simulink model "merginglines"  (R2021a)
settings: Solver=VariableStepAuto  StartTime=0.0  StopTime=10.0  RelTol=1e-3
settings Model: Creator=ibirl  LastModifiedBy=zht

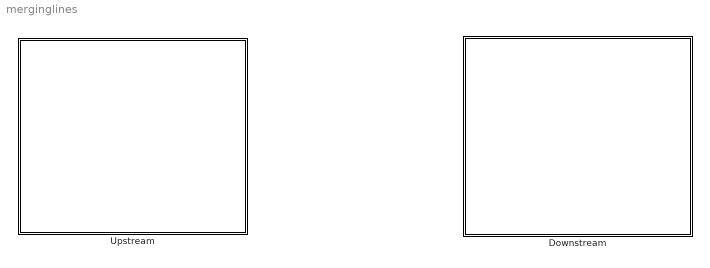
== system merginglines ==
  Downstream : Stateflow chart  TreatAsAtomicUnit=on
  Upstream : Stateflow chart  TreatAsAtomicUnit=on

== stateflow chart merginglines/Downstream ==
  state D1
  state D2
  state D3
  state D4
  D1 -> D1 [order 3] : (1)[1-r3]{0}
  D4 -> D1 [order 2] : (1)[p3]{0}
  D1 -> D3 [order 1] : (1)[r3*pb]{-1}
  D1 -> D2 [order 2] : (1)[r3*(1-pb)]{-1}
  D2 -> D1 [order 2] : (0)[p3*(1-pb)]{0}
  D2 -> D2 [order 3] : (1)[(1-p3)*(1-pb)]{-1}
  D4 -> D2 [order 3] : (1)[(1-p3)*(1-pb)]{-1}
  D2 -> D3 [order 1] : (0)[pb]{-1}
  D3 -> D3 [order 2] : (1)[pbd]{0}
  D3 -> D4 [order 1] : (1)[1-pbd]{0}
  D4 -> D3 [order 1] : (1)[(1-p3)*pb]{-1}

== stateflow chart merginglines/Upstream ==
  state a21
  state a11
  state a31
  state a41
  state a12
  state a22
  state a32
  state a42
  state a33
  state a23
  state a43
  state a13
  state a44
  state a14
  state a24
  state a34
  a41 -> a11 [order 1] : (1)[(p1)*(1-ps1)*(1-r2)]{0}
  a11 -> a31 [order 6] : (1)[r1*ps1*(1-r2)]{1}
  a41 -> a21 [order 5] : (1)[(1-p1)*(1-ps1)*(1-r2)]{1}
  a21 -> a21 [order 5] : (1)[(1-p1)*(1-ps1)*(1-r2)]{1}
  a11 -> a11 [order 1] : (1)[(1-r1)*(1-r2)]{0}
  a21 -> a23 [order 8] : (1)[(1-p1)*(1-ps1)*(r2)*(ps2)]{2}
  a31 -> a31 [order 1] : (1)[(psu1)*(1-r2)]{0}
  a21 -> a11 [order 1] : (1)[p1*(1-ps1)*(1-r2)]{0}
  a21 -> a33 [order 3] : (1)[(1-p1)*ps1*r2*ps2]{2}
  a21 -> a32 [order 9] : (1)[(1-p1)*(ps1)*(r2)*(1-ps2)]{2}
  a21 -> a12 [order 4] : (1)[p1*(1-ps1)*r2*(1-ps2)]{1}
  a22 -> a21 [order 4] : (1)[p1*(1-ps1)*(1-p2)*(1-ps2)]{1}
  a44 -> a11 [order 1] : (1)[(p1)*(1-ps1)*(p2)*(1-ps2)]{0}
  a21 -> a31 [order 7] : (1)[(1-p1)*(ps1)*(1-r2)]{1}
  a31 -> a33 [order 3] : (1)[(psu1)*(r2)*(ps2)]{1}
  a11 -> a21 [order 4] : (1)[r1*(1-ps1)*(1-r2)]{1}
  a14 -> a21 [order 5] : (1)[(r1)*(1-ps1)*(p2)*(1-ps2)]{1}
  a42 -> a21 [order 5] : (1)[(1-p1)*(1-ps1)*(1-r2)]{1}
  a42 -> a11 [order 1] : (1)[(p1)*(1-ps1)*(1-r2)]{0}
  a14 -> a31 [order 7] : (1)[(r1)*(ps1)*(p2)*(1-ps2)]{1}
  a24 -> a31 [order 7] : (1)[(r1)*(ps1)*(p2)*(1-ps2)]{1}
  a44 -> a31 [order 7] : (1)[(1-p1)*(ps1)*(p2)*(1-ps2)]{1}
  a41 -> a23 [order 8] : (1)[(1-p1)*(1-ps1)*(r2)*(ps2)]{2}
  a21 -> a22 [order 2] : (1)[(1-p1)*(1-ps1)*r2*(1-ps2)]{2}
  a12 -> a21 [order 5] : (1)[(r1)*(1-ps1)*(p2)*(1-ps2)]{1}
  a21 -> a13 [order 6] : (1)[(p1)*(1-ps1)*(r2)*(ps2)
      | ]{1}
  a24 -> a21 [order 5] : (1)[(r1)*(1-ps1)*(p2)*(1-ps2)]{1}
  a44 -> a21 [order 5] : (1)[(1-p1)*(1-ps1)*(p2)*(1-ps2)]{1}
  a14 -> a11 [order 1] : (1)[(1-r1)*(p2)*(1-ps2)]{0}
  a31 -> a41 [order 4] : (1)[(1-ppsu1)*(1-r2)]{0}
  a42 -> a31 [order 7] : (1)[(1-p1)*(ps1)*(1-r2)]{1}
  a22 -> a11 [order 1] : (1)[p1*(1-ps1)*p2*(1-ps2)]{0}
  a11 -> a22 [order 2] : (1)[r1*(1-ps1)*r2*(1-ps2)]{2}
  a11 -> a13 [order 5] : (1)[(1-r1)*r2*ps2]{1}
  a24 -> a11 [order 1] : (1)[(1-r1)*(p2)*(1-ps2)]{0}
  a11 -> a12 [order 9] : (1)[(1-r1)*r2*(1-ps2)]{1}
  a11 -> a32 [order 7] : (1)[r1*ps1*r2*(1-ps2)]{2}
  a11 -> a33 [order 3] : (1)[r1*ps1*r2*ps2]{2}
  a11 -> a23 [order 8] : (1)[r1*(1-ps1)*r2*ps2]{2}
  a12 -> a11 [order 1] : (1)[(1-r1)*(p2)*(1-ps2)]{0}
  a12 -> a31 [order 7] : (1)[(r1)*(ps1)*(p2)*(1-ps2)]{1}
  a22 -> a31 [order 8] : (1)[ps1*p2*(1-ps2)]{0}
  a34 -> a31 [order 1] : (1)[(psu1)*(p2)*(1-ps2)]{0}
  a31 -> a42 [order 5] : (1)[(1-ppsu1)*(r2)*(1-ps2)]{1}
  a32 -> a31 [order 1] : (1)[(psu1)*(p2)*(1-ps2)]{0}
  a31 -> a32 [order 2] : (1)[(psu1)*(r2)*(1-ps2)]{1}
  a31 -> a43 [order 6] : (1)[(1-ppsu1)*(r2)*(ps2)]{1}
  a41 -> a31 [order 7] : (1)[(1-p1)*(ps1)*(1-r2)]{1}
  a34 -> a41 [order 4] : (1)[(1-psu1)*(p2)*(1-ps2)]{0}
  a41 -> a12 [order 4] : (1)[(p1)*(1-ps1)*(r2)*(1-ps2)]{1}
  a41 -> a13 [order 6] : (1)[(p1)*(1-ps1)*(r2)*(ps2)]{1}
  a41 -> a22 [order 2] : (1)[(1-p1)*(1-ps1)*(r2)*(1-ps2)]{2}
  a41 -> a33 [order 3] : (1)[(1-p1)*(ps1)*(r2)*(ps2)]{2}
  a32 -> a41 [order 4] : (1)[(1-ppsu1)*(p2)*(1-ps2)]{0}
  a41 -> a32 [order 9] : (1)[(1-p1)*(ps1)*(r2)*(1-ps2)]{2}
  a22 -> a12 [order 5] : (1)[(1-p1)*(1-ps1)*p2*(1-ps2)]{1}
  a12 -> a12 [order 4] : (1)[(1-r1)*(1-p2)*(1-ps2)]{1}
  a12 -> a13 [order 6] : (1)[(1-r1)*(1-p2)*(ps2)]{1}
  a44 -> a12 [order 4] : (1)[(p1)*(1-ps1)*(1-p2)*(1-ps2)]{1}
  a14 -> a12 [order 4] : (1)[(1-r1)*(1-p2)*(1-ps2)]{1}
  a42 -> a22 [order 2] : (1)[(1-p1)*(1-ps1)*(r2)*(1-ps2)]{2}
  a24 -> a12 [order 4] : (1)[(1-r1)*(1-p2)*(1-ps2)]{1}
  a12 -> a33 [order 3] : (1)[(r1)*(ps1)*(1-p2)*(ps2)]{2}
  a12 -> a32 [order 9] : (1)[(r1)*(ps1)*(1-p2)*(1-ps2)]{2}
  a12 -> a22 [order 2] : (1)[(r1)*(1-ps1)*(1-p2)*(1-ps2)]{2}
  a12 -> a23 [order 8] : (1)[(r1)*(1-ps1)*(1-p2)*(ps2)]{2}
  a42 -> a12 [order 4] : (1)[(p1)*(1-ps1)*(r2)*(1-ps2)]{1}
  a32 -> a32 [order 2] : (1)[(psu1)*(1-p2)*(1-ps2)]{1}
  a22 -> a22 [order 2] : (1)[(1-p1)*(1-ps1)*(1-p2)*(1-ps2)]{2}
  a22 -> a32 [order 6] : (1)[ps1*(1-p2)*(1-ps2)]{2}
  a14 -> a22 [order 2] : (1)[(r1)*(1-ps1)*(1-p2)*(1-ps2)]{2}
  a14 -> a32 [order 9] : (1)[(r1)*(ps1)*(1-p2)*(1-ps2)]{2}
  a34 -> a32 [order 2] : (1)[(psu1)*(1-p2)*(1-ps2)]{1}
  a44 -> a32 [order 9] : (1)[(1-p1)*(ps1)*(1-p2)*(1-ps2)]{2}
  a42 -> a13 [order 6] : (1)[(p1)*(1-ps1)*(r2)*(ps2)]{1}
  a22 -> a13 [order 9] : (1)[p1*(1-ps1)*ps2]{0}
  a24 -> a22 [order 2] : (1)[(r1)*(1-ps1)*(1-p2)*(1-ps2)]{2}
  a22 -> a23 [order 7] : (1)[(1-p1)*(1-ps1)*ps2]{2}
  a22 -> a33 [order 3] : (1)[ps1*ps2]{2}
  a44 -> a22 [order 2] : (1)[(1-p1)*(1-ps1)*(1-p2)*(1-ps2)]{2}
  a24 -> a32 [order 9] : (1)[(r1)*(ps1)*(1-p2)*(1-ps2)]{2}
  a42 -> a23 [order 8] : (1)[(1-p1)*(1-ps1)*(r2)*(ps2)]{2}
  a34 -> a42 [order 5] : (1)[(1-psu1)*(1-p2)*(1-ps2)]{1}
  a32 -> a33 [order 3] : (1)[(psu1)*(1-p2)*(ps2)]{1}
  a42 -> a32 [order 9] : (1)[(1-p1)*(ps1)*(r2)*(1-ps2)]{2}
  a32 -> a42 [order 5] : (1)[(1-ppsu1)*(1-p2)*(1-ps2)]{1}
  a32 -> a43 [order 6] : (1)[(1-ppsu1)*(1-p2)*(ps2)]{1}
  a42 -> a33 [order 3] : (1)[(1-p1)*(ps1)*(r2)*(ps2)]{2}
  a43 -> a33 [order 3] : (1)[(1-p1)*(ps1)*(1-psu2)]{0}
  a44 -> a33 [order 3] : (1)[(1-p1)*(ps1)*(1-p2)*(ps2)]{2}
  a33 -> a33 [order 1] : (1)[(psu1)*(psu2)]{0}
  a44 -> a23 [order 8] : (1)[(1-p1)*(1-ps1)*(1-p2)*(ps2)]{2}
  a23 -> a23 [order 2] : (1)[(1-p1)*(1-ps1)*(psu2)]{1}
  a24 -> a33 [order 3] : (1)[(r1)*(ps1)*(1-p2)*(ps2)]{2}
  a33 -> a44 [order 4] : (1)[(1-ppsu1)*(1-ppsu2)]{0}
  a14 -> a23 [order 8] : (1)[(r1)*(1-ps1)*(1-p2)*(ps2)]{2}
  a43 -> a13 [order 1] : (1)[(p1)*(1-ps1)*(psu2)]{0}
  a13 -> a33 [order 3] : (1)[(r1)*(ps1)*(psu2)]{1}
  a14 -> a33 [order 3] : (1)[(r1)*(ps1)*(1-p2)*(ps2)]{2}
  a23 -> a33 [order 3] : (1)[(1-p1)*(ps1)*(psu2)]{1}
  a33 -> a34 [order 2] : (1)[(psu1)*(1-ppsu2)]{0}
  a33 -> a43 [order 3] : (1)[(1-psu1)*(psu2)]{0}
  a34 -> a33 [order 3] : (1)[(psu1)*(1-p2)*(ps2)]{0}
  a43 -> a14 [order 4] : (1)[(p1)*(1-ps1)*(1-psu2)]{0}
  a43 -> a24 [order 5] : (1)[(1-p1)*(1-ps1)*(1-psu2)]{1}
  a43 -> a34 [order 6] : (1)[(1-p1)*(ps1)*(1-psu2)]{1}
  a23 -> a13 [order 1] : (1)[(p1)*(1-ps1)*(psu2)]{0}
  a13 -> a23 [order 2] : (1)[(r1)*(1-ps1)*(psu2)]{1}
  a23 -> a14 [order 4] : (1)[(p1)*(1-ps1)*(1-ppsu2)]{0}
  a24 -> a23 [order 8] : (1)[(r1)*(1-ps1)*(1-p2)*(ps2)]{2}
  a23 -> a24 [order 5] : (1)[(1-p1)*(1-ps1)*(1-ppsu2)]{1}
  a23 -> a34 [order 6] : (1)[(1-p1)*(ps1)*(1-ppsu2)]{1}
  a43 -> a23 [order 2] : (1)[(1-p1)*(1-ps1)*(psu2)]{1}
  a34 -> a43 [order 6] : (1)[(1-psu1)*(1-p2)*(ps2)]{1}
  a14 -> a13 [order 6] : (1)[(1-r1)*(1-p2)*(ps2)]{1}
  a44 -> a13 [order 6] : (1)[(1-p1)*(1-ps1)*(1-p2)*(ps2)]{1}
  a13 -> a13 [order 1] : (1)[(1-r1)*(psu2)]{0}
  a13 -> a14 [order 4] : (1)[(1-r1)*(1-ppsu2)]{0}
  a24 -> a13 [order 6] : (1)[(1-r1)*(1-p2)*(ps2)]{1}
  a13 -> a24 [order 5] : (1)[(r1)*(1-ps1)*(1-ppsu2)]{1}
  a13 -> a34 [order 6] : (1)[(r1)*(ps1)*(1-ppsu2)]{1}
